simulink subsystem "Motion_Sim"  (R2020a)
settings: Solver=VariableStepAuto  StartTime=0.0  StopTime=10.0  RelTol=1e-3
undefined symbols (not defined in the file or in its folder): initX, initY, initYaw
libraries: simulink_extras x1, simulink x1
settings Model: Creator=Duncan  LastModifiedBy=abatra2

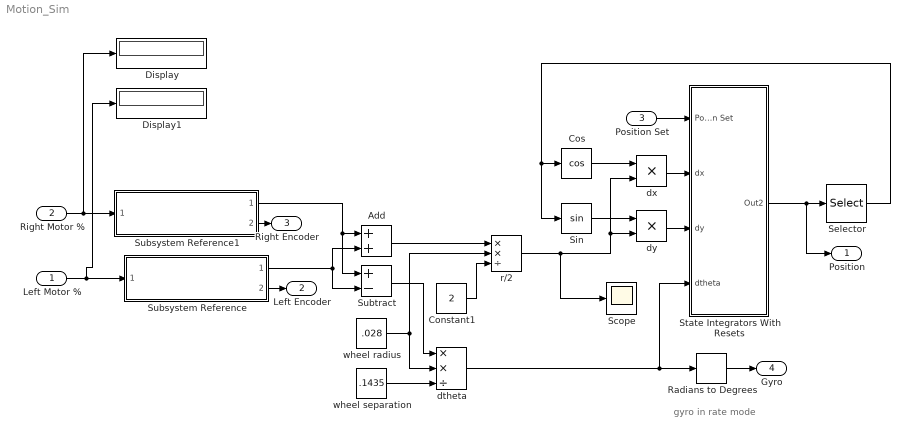
== system Motion_Sim ==
  note: gyro in rate mode
  Left Motor % : Inport
  Right Motor % : Inport  Port=2
  Position Set : Inport  Port=3
  Add : Sum
  Constant1 : Constant  Value=2
  Cos : Trigonometry  Operator=cos
  Display : Display
  Display1 : Display
  Radians to Degrees : simulink_extras/Transformations/Radians to Degrees
  Scope : Scope
  Selector : Selector  InputPortWidth=3  IndexOptions=Index vector (dialog)  Indices=3  OutputSizes=1
  Sin : Trigonometry
  State Integrators With Resets : Subsystem
  Subsystem Reference : Subsystem  ReferencedSubsystem=LegoMotor  ResetMode=Reset at each sample time
  Subsystem Reference1 : Subsystem  ReferencedSubsystem=LegoMotor  ResetMode=Reset at each sample time
  Subtract : Sum  Inputs=+-
  dtheta : Product  Inputs=**/
  dx : Product  Inputs=**
  dy : Product  Inputs=**
  r/2 : Product  Inputs=**/
  wheel radius : Constant  Value=.028
  wheel separation : Constant  Value=.1435
  Position : Outport
  Left Encoder : Outport  Port=2
  Right Encoder : Outport  Port=3
  Gyro : Outport  Port=4
  wires:
  Right Motor %/1 -> Display/1, Subsystem Reference1/1
  Subsystem Reference/1 -> Add/2, Subtract/2
  Subsystem Reference/2 -> Left Encoder/1
  Left Motor %/1 -> Display1/1, Subsystem Reference/1
  Subsystem Reference1/1 -> Subtract/1, Add/1
  Subsystem Reference1/2 -> Right Encoder/1
  Selector/1 -> Sin/1, Cos/1
  State Integrators With Resets/1(Out2) -> Position/1, Selector/1
  dy/1 -> State Integrators With Resets/3(dy)
  dx/1 -> State Integrators With Resets/2(dx)
  Position Set/1 -> State Integrators With Resets/1(Position Set)
  r/2/1 -> dy/2, dx/2, Scope/1
  Sin/1 -> dy/1
  Cos/1 -> dx/1
  Add/1 -> r/2/1
  Constant1/1 -> r/2/3
  Radians to Degrees/1 -> Gyro/1
  dtheta/1 -> Radians to Degrees/1, State Integrators With Resets/4(dtheta)
  Subtract/1 -> dtheta/1
  wheel separation/1 -> dtheta/3
  wheel radius/1 -> dtheta/2, r/2/2

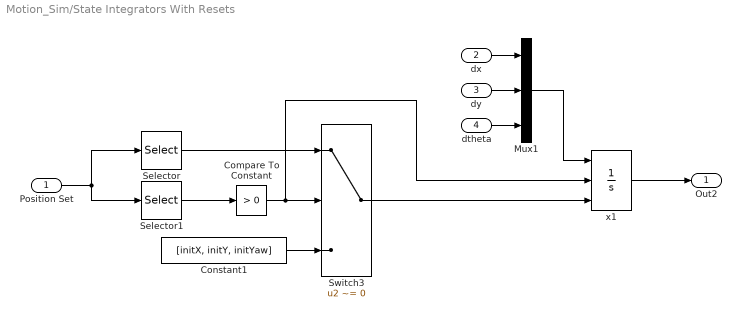
== system Motion_Sim/State Integrators With Resets ==
  Position Set : Inport
  dx : Inport  Port=2
  dy : Inport  Port=3
  dtheta : Inport  Port=4
  Compare To Constant : simulink/Logic and Bit Operations/Compare To Constant  relop=>  const=0  OutDataTypeStr=boolean
  Constant1 : Constant  Value=[initX, initY, initYaw]
  Mux1 : Mux  Inputs=3
  Selector : Selector  InputPortWidth=4  IndexOptions=Index vector (dialog)  Indices=[2:4]  OutputSizes=1
  Selector1 : Selector  InputPortWidth=4  IndexOptions=Index vector (dialog)  Indices=1  OutputSizes=1
  Switch3 : Switch  Criteria=u2 ~= 0
  x1 : Integrator  ExternalReset=rising  InitialConditionSource=external  InitialCondition=initX
  Out2 : Outport
  wires:
  Position Set/1 -> Selector1/1, Selector/1
  Compare To Constant/1 -> x1/2, Switch3/2
  Selector1/1 -> Compare To Constant/1
  dy/1 -> Mux1/2
  dtheta/1 -> Mux1/3
  dx/1 -> Mux1/1
  Selector/1 -> Switch3/1
  Constant1/1 -> Switch3/3
  Switch3/1 -> x1/3
  Mux1/1 -> x1/1
  x1/1 -> Out2/1
